simulink model "week1_problem10"  (R2020b)
settings: Solver=VariableStepAuto  StartTime=0.0  StopTime=10.0  RelTol=1e-3
settings Model: Creator=gauri  LastModifiedBy=mluser

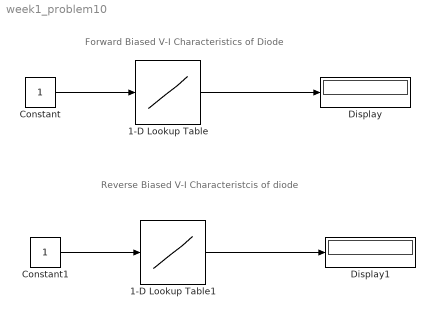
== system week1_problem10 ==
  note: Reverse Biased V-I Characteristcis of diode
  note: Forward Biased V-I Characteristics of Diode
  1-D Lookup Table : Lookup_n-D  NumberOfTableDimensions=1  BreakpointsForDimension1=|  Table=|  InternalRulePriority=Speed  RndMeth=Simplest  InputSameDT=on
      BreakpointsForDimension1=|
      | [0.283
      | 0.347
      | 0.37
      | 0.395
      | 0.425
      | 0.435
      | 0.445
      | 0.467
      | 0.485
      | 0.496
      | 0.503
      | 0.517
      | 0.525
      | 0.527
      | 0.538
      | 0.544
      | 0.555
      | 0.563
      | 0.573
      | 0.575
      | 0.585
      | 0.592
      | 0.598
      | 0.605
      | 0.618
      | 0.623
      | 0.63
      | 0.646
      | 0.653
      | 0.658
      | 0.665
      | 0.672
      | 0.677
      | 0.68
      | ]
      Table=|
      | [0
      | 0.001
      | 0.001
      | 0.005
      | 0.009
      | 0.012
      | 0.018
      | 0.047
      | 0.06
      | 0.082
      | 0.101
      | 0.145
      | 0.175
      | 0.181
      | 0.246
      | 0.306
      | 0.412
      | 0.509
      | 0.646
      | 0.693
      | 0.822
      | 0.979
      | 1.112
      | 1.335
      | 1.805
      | 2.007
      | 2.392
      | 3.4
      | 3.9
      | 4.3
      | 5.3
      | 6.7
      | 7.6
      | 8
      | ]
  1-D Lookup Table1 : Lookup_n-D  NumberOfTableDimensions=1  BreakpointsForDimension1=|  Table=|  InternalRulePriority=Speed  RndMeth=Simplest  InputSameDT=on
      BreakpointsForDimension1=|
      | [0.9
      | 1.6
      | 2.07
      | 3.78
      | 4.94
      | 5.95
      | 7.27
      | 8.01
      | 9.32
      | 9.84
      | 10.34
      | 11.94
      | 12.77
      | 13.93
      | 15.11
      | 16.32
      | 17.03
      | 17.81
      | 18.56
      | 19.35
      | ]
      Table=|
      | [0
      | 0.001
      | 0.002
      | 0.003
      | 0.004
      | 0.005
      | 0.006
      | 0.007
      | 0.008
      | 0.009
      | 0.01
      | 0.011
      | 0.012
      | 0.013
      | 0.014
      | 0.015
      | 0.016
      | 0.017
      | 0.018
      | 0.019
      | ]
  Constant : Constant
  Constant1 : Constant
  Display : Display
  Display1 : Display
  wires:
  Constant/1 -> 1-D Lookup Table/1
  1-D Lookup Table/1 -> Display/1
  1-D Lookup Table1/1 -> Display1/1
  Constant1/1 -> 1-D Lookup Table1/1
